simulink model "Gearshift"  (R2025b)
settings: Solver=FixedStepAuto  StartTime=0.0  StopTime=10.0  FixedStep=0.01  RelTol=1e-3  EnableMultiTasking=on
undefined symbols (not defined in the file): downtab, uptab
settings Model: DataDictionary=myNewDictionary.sldd  Creator=yoyuan  LastModifiedBy=yoyuan
settings SolverCC: AlgebraicLoopSolver=TrustRegion  AutoInsertRateTranBlk=on
settings DataIOCC: LimitDataPoints=on
settings OptimizationCC: LifeSpan=inf
settings DebuggingCC: UnconnectedInputMsg=warning  UnconnectedOutputMsg=warning  UnconnectedLineMsg=warning  AllowSymbolicDim=off  SFUnexpectedBacktrackingDiag=warning  SFNoUnconditionalDefaultTransitionDiag=warning  SFExecutionAtInitializationDiag=none  ArithmeticOperatorsInVariantConditions=warning
settings ModelReferenceCC: EnableRefExpFcnMdlSchedulingChecks=on
settings SFSimCC: SimUseLocalCustomCode=off  CustomCodeUndefinedFunction=UseInterfaceOnly
settings RTWCC: RTWUseLocalCustomCode=off  GPUComputeCapability=3.5  DLArmComputeVersion=19.05
settings CodeAppCC: StateflowObjectComments=on
settings GRTTargetCC: TargetLangStandard=C89/C90 (ANSI)
settings ConfigComp: CovMetricSettings=dw  CovSaveCumulativeToWorkspaceVar=on  CovSaveSingleToWorkspaceVar=on  CovExternalEMLEnable=off  CovSFcnEnable=off

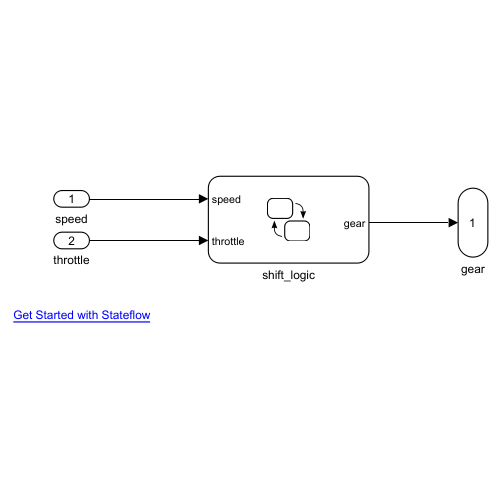
[thumbnail: Simulink's stored preview of the top-level diagram]
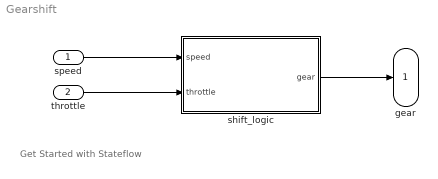
== system Gearshift ==
  note: Get Started with Stateflow
  speed : Inport
  throttle : Inport  Port=2
  shift_logic : Stateflow chart  TreatAsAtomicUnit=on
  gear : Outport
  wires:
  speed/1 -> shift_logic/1(speed)
  throttle/1 -> shift_logic/2(throttle)
  shift_logic/1(gear) -> gear/1

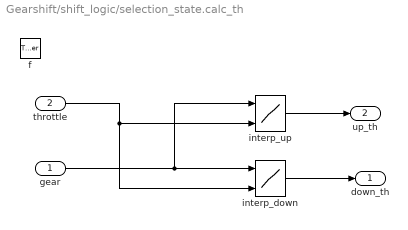
== system Gearshift/shift_logic/selection_state.calc_th ==
  gear : Inport
  throttle : Inport  Port=2
  f : TriggerPort  TriggerType=function-call  VariantControl=(inherit)
      settings: CopyFcn=Stateflow.SLINSF.SimulinkMan.removeBlockPreDeleteFcn  PreDeleteFcn=Stateflow.SLINSF.SimulinkMan.unsafePredeleteFcn
  interp_down : Lookup2D  RowIndex=downth  ColumnIndex=[1:4]  Table=downtab  SaturateOnIntegerOverflow=off
  interp_up : Lookup2D  RowIndex=upth  ColumnIndex=[1:4]  Table=uptab  SaturateOnIntegerOverflow=off
  down_th : Outport  VectorParamsAs1DForOutWhenUnconnected=off
  up_th : Outport  Port=2  VectorParamsAs1DForOutWhenUnconnected=off
  wires:
  interp_up/1 -> up_th/1
  interp_down/1 -> down_th/1
  throttle/1 -> interp_down/2, interp_up/2
  gear/1 -> interp_down/1, interp_up/1

== stateflow chart Gearshift/shift_logic ==
  settings: updateMethod=DISCRETE  sampleTime=0.04
  state gear_state [parallel]
    settings: executionOrder=1
    state fourth
      entry: gear = 4;
    state third
      entry: gear = 3;
    state second
      entry: gear = 2;
    state first
      entry: gear = 1;
    (default) -> first
    second -> third [order 1] : UP
    first -> second : UP
    third -> fourth [order 1] : UP
    third -> second [order 2] : DOWN
    fourth -> third [order 2] : DOWN
    second -> first [order 2] : DOWN
    fourth -> second [order 1] : KICKDOWN
  state selection_state [parallel]
    during: [down_th,up_th] = calc_th(gear,throttle);
    settings: executionOrder=2
    state steady_state
    state downshifting
    state upshifting
    state kickdown
    state [down_th,up_th] = calc_th(gear,throttle) [function]
    (default) -> steady_state
    steady_state -> (junction 43) [order 2] : [speed < down_th]
    steady_state -> upshifting [order 1] : [speed > up_th]
    (junction 43) -> kickdown [order 1] : [gear==4 && throttle > 96]
    kickdown -> steady_state [order 2] : [speed > down_th]
    kickdown -> steady_state [order 1] : after(TWAIT,tick)
        | [speed >= up_th]
        | {gear_state.KICKDOWN;}
    downshifting -> steady_state [order 1] : after(TWAIT,tick)
        | [speed <= down_th]
        | {gear_state.DOWN;}
    downshifting -> steady_state [order 2] : [speed > down_th]
    upshifting -> steady_state [order 1] : after(TWAIT,tick)
        | [speed >= up_th]
        | {gear_state.UP;}
    upshifting -> steady_state [order 2] : [speed < up_th]
    (junction 43) -> downshifting [order 2]
  data: gear function_input; throttle function_input; down_th function_output; up_th function_output; speed input double; gear output double [1..4]; TWAIT parameter uint8; up_th local double; down_th local double; throttle input
  events: DOWN local EITHER_EDGE_EVENT; UP local EITHER_EDGE_EVENT; KICKDOWN local FUNCTION_CALL_EVENT
